simulink model "RL_SAC"  (R2025a)
settings: Solver=FixedStepDiscrete  StartTime=0.0  StopTime=20  FixedStep=1e-2  RelTol=1e-6
undefined symbols (not defined in the file or in its folder): DiscIntNeverNeededParam
libraries: simulink x26, cstblocks x16, slpidlib x2, aerolibutil x2, rllib x1
(part 2 of 2)

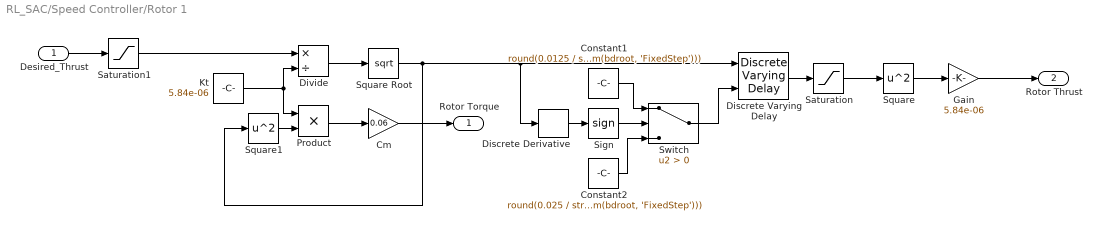
== system RL_SAC/Speed Controller/Rotor 1 ==
  Desired_Thrust : Inport
  Cm : Gain  Gain=0.06
  Constant1 : Constant  Value=round(0.0125 / str2double(get_param(bdroot, 'FixedStep')))
  Constant2 : Constant  Value=round(0.025 / str2double(get_param(bdroot, 'FixedStep')))
  Discrete Derivative : simulink/Discrete/Discrete Derivative  gainval=1.0  ICPrevScaledInput=0.0  OutMin=[]  OutMax=[]  OutDataType=fixdt(1, 16)  OutScaling=2^-10  DoSatur=off
  Discrete Varying Delay : cstblocks/Linear Parameter Varying/Discrete Varying Delay  Td=1  TdMax=10  TdFixed=[]  u0=0  Ts=-1  PreventDirectFeedthrough=off
  Divide : Product  Inputs=*/
  Gain : Gain  Gain=5.84e-06
  Kt : Constant  Value=5.84e-06
  Product : Product
  Saturation : Saturate  UpperLimit=1100  LowerLimit=0
  Saturation1 : Saturate  UpperLimit=inf  LowerLimit=0
  Sign : Signum
  Square : Math  Operator=square
  Square Root : Sqrt
  Square1 : Math  Operator=square
  Switch : Switch  Criteria=u2 > Threshold  SaturateOnIntegerOverflow=off  InputSameDT=off
  Rotor Torque : Outport
  Rotor Thrust : Outport  Port=2
  wires:
  Desired_Thrust/1 -> Saturation1/1
  Saturation/1 -> Square/1
  Switch/1 -> Discrete Varying Delay/2
  Constant2/1 -> Switch/3
  Discrete Varying Delay/1 -> Saturation/1
  Discrete Derivative/1 -> Sign/1
  Constant1/1 -> Switch/1
  Square Root/1 -> Discrete Varying Delay/1, Discrete Derivative/1, Square1/1
  Sign/1 -> Switch/2
  Square/1 -> Gain/1
  Kt/1 -> Divide/2, Product/1
  Divide/1 -> Square Root/1
  Product/1 -> Cm/1
  Square1/1 -> Product/2
  Cm/1 -> Rotor Torque/1
  Gain/1 -> Rotor Thrust/1
  Saturation1/1 -> Divide/1

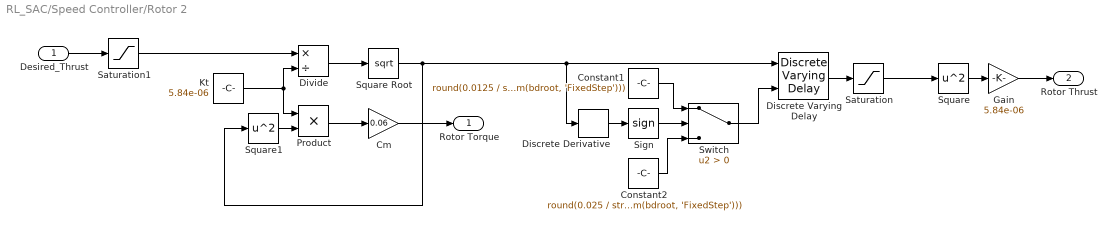
== system RL_SAC/Speed Controller/Rotor 2 ==
  Desired_Thrust : Inport
  Cm : Gain  Gain=0.06
  Constant1 : Constant  Value=round(0.0125 / str2double(get_param(bdroot, 'FixedStep')))
  Constant2 : Constant  Value=round(0.025 / str2double(get_param(bdroot, 'FixedStep')))
  Discrete Derivative : simulink/Discrete/Discrete Derivative  gainval=1.0  ICPrevScaledInput=0.0  OutMin=[]  OutMax=[]  OutDataType=fixdt(1, 16)  OutScaling=2^-10  DoSatur=off
  Discrete Varying Delay : cstblocks/Linear Parameter Varying/Discrete Varying Delay  Td=1  TdMax=10  TdFixed=[]  u0=0  Ts=-1  PreventDirectFeedthrough=off
  Divide : Product  Inputs=*/
  Gain : Gain  Gain=5.84e-06
  Kt : Constant  Value=5.84e-06
  Product : Product
  Saturation : Saturate  UpperLimit=1100  LowerLimit=0
  Saturation1 : Saturate  UpperLimit=inf  LowerLimit=0
  Sign : Signum
  Square : Math  Operator=square
  Square Root : Sqrt
  Square1 : Math  Operator=square
  Switch : Switch  Criteria=u2 > Threshold  SaturateOnIntegerOverflow=off  InputSameDT=off
  Rotor Torque : Outport
  Rotor Thrust : Outport  Port=2
  wires:
  Cm/1 -> Rotor Torque/1
  Square1/1 -> Product/2
  Product/1 -> Cm/1
  Divide/1 -> Square Root/1
  Kt/1 -> Product/1, Divide/2
  Saturation1/1 -> Divide/1
  Gain/1 -> Rotor Thrust/1
  Square/1 -> Gain/1
  Sign/1 -> Switch/2
  Square Root/1 -> Square1/1, Discrete Derivative/1, Discrete Varying Delay/1
  Constant1/1 -> Switch/1
  Discrete Derivative/1 -> Sign/1
  Discrete Varying Delay/1 -> Saturation/1
  Constant2/1 -> Switch/3
  Switch/1 -> Discrete Varying Delay/2
  Saturation/1 -> Square/1
  Desired_Thrust/1 -> Saturation1/1

== system RL_SAC/Speed Controller/Rotor 3 ==
  Desired_Thrust : Inport
  Cm : Gain  Gain=0.06
  Constant1 : Constant  Value=round(0.0125 / str2double(get_param(bdroot, 'FixedStep')))
  Constant2 : Constant  Value=round(0.025 / str2double(get_param(bdroot, 'FixedStep')))
  Discrete Derivative : simulink/Discrete/Discrete Derivative  gainval=1.0  ICPrevScaledInput=0.0  OutMin=[]  OutMax=[]  OutDataType=fixdt(1, 16)  OutScaling=2^-10  DoSatur=off
  Discrete Varying Delay : cstblocks/Linear Parameter Varying/Discrete Varying Delay  Td=1  TdMax=10  TdFixed=[]  u0=0  Ts=-1  PreventDirectFeedthrough=off
  Divide : Product  Inputs=*/
  Gain : Gain  Gain=5.84e-06
  Kt : Constant  Value=5.84e-06
  Product : Product
  Saturation : Saturate  UpperLimit=1100  LowerLimit=0
  Saturation1 : Saturate  UpperLimit=inf  LowerLimit=0
  Sign : Signum
  Square : Math  Operator=square
  Square Root : Sqrt
  Square1 : Math  Operator=square
  Switch : Switch  Criteria=u2 > Threshold  SaturateOnIntegerOverflow=off  InputSameDT=off
  Rotor Torque : Outport
  Rotor Thrust : Outport  Port=2
  wires:
  Desired_Thrust/1 -> Saturation1/1
  Saturation/1 -> Square/1
  Switch/1 -> Discrete Varying Delay/2
  Constant2/1 -> Switch/3
  Discrete Varying Delay/1 -> Saturation/1
  Discrete Derivative/1 -> Sign/1
  Constant1/1 -> Switch/1
  Square Root/1 -> Discrete Varying Delay/1, Discrete Derivative/1, Square1/1
  Sign/1 -> Switch/2
  Square/1 -> Gain/1
  Gain/1 -> Rotor Thrust/1
  Saturation1/1 -> Divide/1
  Kt/1 -> Divide/2, Product/1
  Divide/1 -> Square Root/1
  Product/1 -> Cm/1
  Square1/1 -> Product/2
  Cm/1 -> Rotor Torque/1

== system RL_SAC/Speed Controller/Rotor 4 ==
  Desired_Thrust : Inport
  Cm : Gain  Gain=0.06
  Constant1 : Constant  Value=round(0.0125 / str2double(get_param(bdroot, 'FixedStep')))
  Constant2 : Constant  Value=round(0.025 / str2double(get_param(bdroot, 'FixedStep')))
  Discrete Derivative : simulink/Discrete/Discrete Derivative  gainval=1.0  ICPrevScaledInput=0.0  OutMin=[]  OutMax=[]  OutDataType=fixdt(1, 16)  OutScaling=2^-10  DoSatur=off
  Discrete Varying Delay : cstblocks/Linear Parameter Varying/Discrete Varying Delay  Td=1  TdMax=10  TdFixed=[]  u0=0  Ts=-1  PreventDirectFeedthrough=off
  Divide : Product  Inputs=*/
  Gain : Gain  Gain=5.84e-06
  Kt : Constant  Value=5.84e-06
  Product : Product
  Saturation : Saturate  UpperLimit=1100  LowerLimit=0
  Saturation1 : Saturate  UpperLimit=inf  LowerLimit=0
  Sign : Signum
  Square : Math  Operator=square
  Square Root : Sqrt
  Square1 : Math  Operator=square
  Switch : Switch  Criteria=u2 > Threshold  SaturateOnIntegerOverflow=off  InputSameDT=off
  Rotor Torque : Outport
  Rotor Thrust : Outport  Port=2
  wires:
  Cm/1 -> Rotor Torque/1
  Square1/1 -> Product/2
  Product/1 -> Cm/1
  Divide/1 -> Square Root/1
  Kt/1 -> Product/1, Divide/2
  Saturation1/1 -> Divide/1
  Gain/1 -> Rotor Thrust/1
  Square/1 -> Gain/1
  Sign/1 -> Switch/2
  Square Root/1 -> Square1/1, Discrete Derivative/1, Discrete Varying Delay/1
  Constant1/1 -> Switch/1
  Discrete Derivative/1 -> Sign/1
  Discrete Varying Delay/1 -> Saturation/1
  Constant2/1 -> Switch/3
  Switch/1 -> Discrete Varying Delay/2
  Saturation/1 -> Square/1
  Desired_Thrust/1 -> Saturation1/1

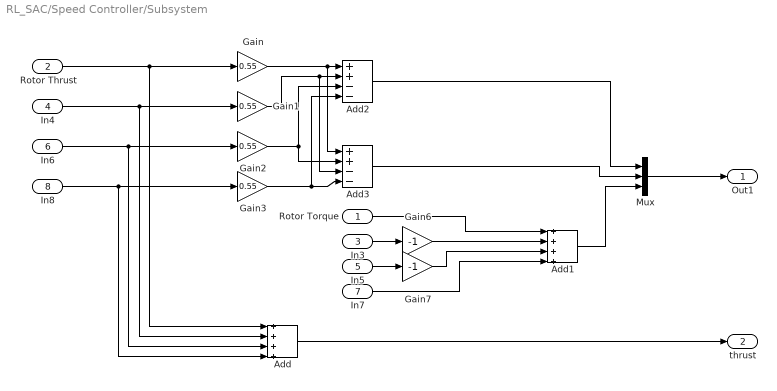
== system RL_SAC/Speed Controller/Subsystem ==
  Rotor Torque : Inport
  Rotor Thrust : Inport  Port=2
  In3 : Inport  Port=3
  In4 : Inport  Port=4
  In5 : Inport  Port=5
  In6 : Inport  Port=6
  In7 : Inport  Port=7
  In8 : Inport  Port=8
  Add : Sum  Inputs=++++
  Add1 : Sum  Inputs=++++
  Add2 : Sum  Inputs=++--
  Add3 : Sum  Inputs=++--
  Gain{,1..3} (4 alike) : Gain  Gain=0.55
  Gain6 : Gain  Gain=-1
  Gain7 : Gain  Gain=-1
  Mux : Mux  Inputs=3
  Out1 : Outport
  thrust : Outport  Port=2
  wires:
  Mux/1 -> Out1/1
  Add/1 -> thrust/1
  Add2/1 -> Mux/1
  Add3/1 -> Mux/2
  Add1/1 -> Mux/3
  In7/1 -> Add1/4
  In3/1 -> Gain6/1
  Rotor Torque/1 -> Add1/1
  In8/1 -> Gain3/1, Add/4
  Rotor Thrust/1 -> Gain/1, Add/1
  Gain/1 -> Add3/1, Add2/1
  Gain1/1 -> Add3/3, Add2/2
  Gain2/1 -> Add2/3, Add3/2
  Gain3/1 -> Add3/4, Add2/4
  In4/1 -> Add/2, Gain1/1
  In6/1 -> Add/3, Gain2/1
  Gain6/1 -> Add1/2
  In5/1 -> Gain7/1
  Gain7/1 -> Add1/3

== system RL_SAC/Attitude Control/RL/disturbance ==
  In1 : Inport
  DistDur : Inport  Port=2
  Add : Sum
  Add1 : Sum
  Constant : Constant  Value=6
  Delay : Delay  DelayLength=200
  Gain : Gain  Gain=-1
  Variable Time Delay : VariableTransportDelay  MaximumDelay=14  MaximumPoints=2048
  u : Outport
  wires:
  Gain/1 -> Variable Time Delay/1
  Delay/1 -> Add/1
  Variable Time Delay/1 -> Add/2
  In1/1 -> Delay/1, Gain/1
  Add/1 -> u/1
  Constant/1 -> Add1/2
  Add1/1 -> Variable Time Delay/2
  DistDur/1 -> Add1/1

== system RL_SAC/Attitude Control/RL/disturbance1 ==
  In1 : Inport
  DistDur : Inport  Port=2
  Add : Sum
  Add1 : Sum
  Constant : Constant  Value=2
  Delay : Delay  DelayLength=200
  Gain : Gain  Gain=-1
  Variable Time Delay : VariableTransportDelay  MaximumDelay=14  MaximumPoints=2048
  u : Outport
  wires:
  Add/1 -> u/1
  In1/1 -> Delay/1, Gain/1
  Variable Time Delay/1 -> Add/2
  Delay/1 -> Add/1
  Gain/1 -> Variable Time Delay/1
  Constant/1 -> Add1/2
  Add1/1 -> Variable Time Delay/2
  DistDur/1 -> Add1/1

== system RL_SAC/Attitude Control/RL/observation ==
  F_A_Pos : Inport
  b a vel : Inport  Port=2
  pos_error : Inport  Port=3
  DistDur : Inport  Port=4
  wind : Inport  Port=5
  Abs1 : Abs  SaturateOnIntegerOverflow=off
  Compare To Constant1 : simulink/Logic and Bit Operations/Compare To Constant  relop=>=  const=0.1  OutDataTypeStr=boolean
  Constant1 : Constant
  Data Type Conversion : DataTypeConversion  OutDataTypeStr=double  SaturateOnIntegerOverflow=off  RndMeth=Floor
  Mux : Mux  Inputs=5
  Selector2 : Selector  InputPortWidth=3  IndexOptions=Index vector (dialog)  Indices=[1]  OutputSizes=1
  disturbance1 : Subsystem
      settings: PortSchema="{\"entries\":[{\"content\":{\"sides\":[{\"content\":{\"connectorIds\":[\"In1\"]},\"type\":\"ConnectorPlacement.EquallySpacedRectSide\",\"uuid\":\"1ea45d97-72cc-4587-9cbf-0adeb2cc8bb7\"},{\"content\":{\"connectorIds\":[\"Out1\"],\"side\":\"RIGHT\"},\"type\":\"ConnectorPlacement.EquallySpacedRectSide\",\"uuid\":\"61165e1b-28cc-48e7-99ef-5ed7ad2a03a2\"},{\"content\":{\"side\":\"TOP\"},\"type\":\"ConnectorPlacement.EquallySpacedRectSide\",\"uuid\":\"1ee858fb-66c9-4560-b1d5-e0dc7ce4c9ca\"},{\"content\":{\"connectorIds\":[\"In2\"],\"side\":\"BOTTOM\"},\"type\":\"ConnectorPlacement.EquallySpacedRectSide\",\"uuid\":\"8aed40e2-8781-4923-8805-61cf0e1b563e\"}]},\"type\":\"ConnectorPlacement.EquallySpacedConnector\",\"uuid\":\"317ef023-ce87-4b82-add9-53b7146a0621\"}],\"packageUris\":[\"http://schema.mathworks.com/mf0/Connector/R2020b\"],\"version\":\"1.0\"}"
  Out1 : Outport
  wires:
  F_A_Pos/1 -> Selector2/1
  Abs1/1 -> Compare To Constant1/1
  Compare To Constant1/1 -> Data Type Conversion/1
  Data Type Conversion/1 -> Mux/2
  Mux/1 -> Out1/1
  Constant1/1 -> disturbance1/1(In1)
  disturbance1/1(u) -> Abs1/1
  DistDur/1 -> disturbance1/2(DistDur)
  wind/1 -> Mux/1
  Selector2/1 -> Mux/3
  b a vel/1 -> Mux/4
  pos_error/1 -> Mux/5

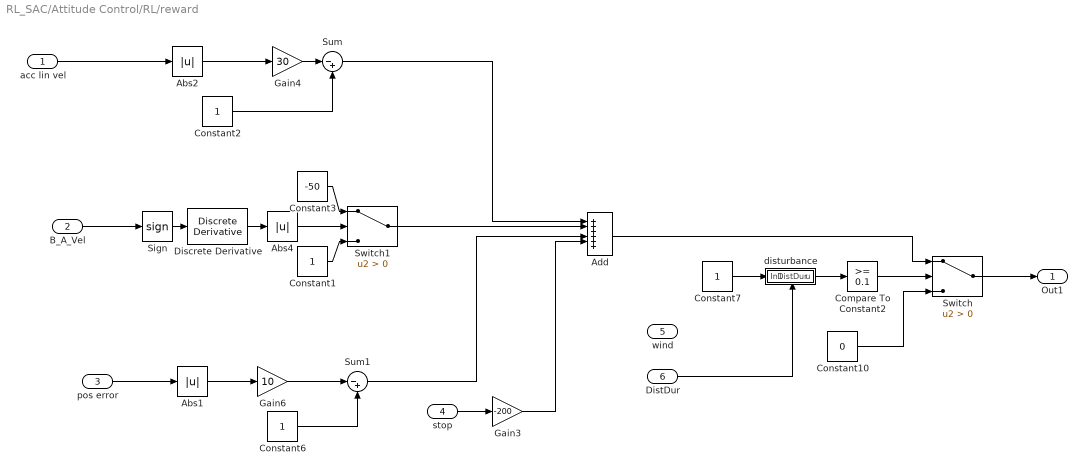
== system RL_SAC/Attitude Control/RL/reward ==
  acc lin vel : Inport
  B_A_Vel : Inport  Port=2
  pos error : Inport  Port=3
  stop : Inport  Port=4
  wind : Inport  Port=5
  DistDur : Inport  Port=6
  Abs1 : Abs  SaturateOnIntegerOverflow=off
  Abs2 : Abs  SaturateOnIntegerOverflow=off
  Abs4 : Abs  SaturateOnIntegerOverflow=off
  Add : Sum  Inputs=++++++
  Compare To Constant2 : simulink/Logic and Bit Operations/Compare To Constant  relop=>=  const=0.1  OutDataTypeStr=boolean
  Constant{1..2,6..7} (4 alike) : Constant
  Constant10 : Constant  Value=0
  Constant3 : Constant  Value=-50
  Discrete Derivative : simulink/Discrete/Discrete Derivative  gainval=1.0  ICPrevScaledInput=0.0  OutMin=[]  OutMax=[]  OutDataType=fixdt(1, 16)  OutScaling=2^-10  DoSatur=off
  Gain3 : Gain  Gain=-200
  Gain4 : Gain  Gain=30
  Gain6 : Gain  Gain=10
  Sign : Signum
  Sum : Sum  Inputs=|-+
  Sum1 : Sum  Inputs=|-+
  Switch : Switch  Criteria=u2 > Threshold  SaturateOnIntegerOverflow=off  InputSameDT=off
  Switch1 : Switch  Criteria=u2 > Threshold  SaturateOnIntegerOverflow=off  InputSameDT=off
  disturbance : Subsystem
      settings: PortSchema="{\"entries\":[{\"content\":{\"sides\":[{\"content\":{\"connectorIds\":[\"In1\"]},\"type\":\"ConnectorPlacement.EquallySpacedRectSide\",\"uuid\":\"1ea45d97-72cc-4587-9cbf-0adeb2cc8bb7\"},{\"content\":{\"connectorIds\":[\"Out1\"],\"side\":\"RIGHT\"},\"type\":\"ConnectorPlacement.EquallySpacedRectSide\",\"uuid\":\"61165e1b-28cc-48e7-99ef-5ed7ad2a03a2\"},{\"content\":{\"side\":\"TOP\"},\"type\":\"ConnectorPlacement.EquallySpacedRectSide\",\"uuid\":\"1ee858fb-66c9-4560-b1d5-e0dc7ce4c9ca\"},{\"content\":{\"connectorIds\":[\"In2\"],\"side\":\"BOTTOM\"},\"type\":\"ConnectorPlacement.EquallySpacedRectSide\",\"uuid\":\"88debdfa-6370-4c36-898f-2948795f08ca\"}]},\"type\":\"ConnectorPlacement.EquallySpacedConnector\",\"uuid\":\"317ef023-ce87-4b82-add9-53b7146a0621\"}],\"packageUris\":[\"http://schema.mathworks.com/mf0/Connector/R2020b\"],\"version\":\"1.0\"}"
  Out1 : Outport
  wires:
  Abs2/1 -> Gain4/1
  Constant10/1 -> Switch/3
  Abs1/1 -> Gain6/1
  stop/1 -> Gain3/1
  Sign/1 -> Discrete Derivative/1
  Discrete Derivative/1 -> Abs4/1
  Abs4/1 -> Switch1/2
  Constant1/1 -> Switch1/3
  Constant3/1 -> Switch1/1
  Switch1/1 -> Add/2
  Gain3/1 -> Add/5
  B_A_Vel/1 -> Sign/1
  Constant7/1 -> disturbance/1(In1)
  disturbance/1(u) -> Compare To Constant2/1
  Compare To Constant2/1 -> Switch/2
  Add/1 -> Switch/1
  Switch/1 -> Out1/1
  pos error/1 -> Abs1/1
  acc lin vel/1 -> Abs2/1
  Gain4/1 -> Sum/1
  Constant2/1 -> Sum/2
  Sum/1 -> Add/1
  Gain6/1 -> Sum1/1
  Sum1/1 -> Add/4
  Constant6/1 -> Sum1/2
  DistDur/1 -> disturbance/2(DistDur)

== system RL_SAC/Attitude Control/RL/stop ==
  pos error : Inport
  F_A_Pos : Inport  Port=2
  B_A_Vel : Inport  Port=3
  wind : Inport  Port=4
  DistDur : Inport  Port=5
  AND1 : Logic  IconShape=distinctive  AllPortsSameDT=off  OutDataTypeStr=boolean
  Abs : Abs  SaturateOnIntegerOverflow=off
  Abs2 : Abs  SaturateOnIntegerOverflow=off
  Abs3 : Abs  SaturateOnIntegerOverflow=off
  Compare To Constant : simulink/Logic and Bit Operations/Compare To Constant  relop=>=  const=2  OutDataTypeStr=boolean
  Compare To Constant1 : simulink/Logic and Bit Operations/Compare To Constant  relop=>=  const=0.1  OutDataTypeStr=boolean
  Compare To Constant2 : simulink/Logic and Bit Operations/Compare To Constant  relop=>=  const=2  OutDataTypeStr=boolean
  Compare To Constant3 : simulink/Logic and Bit Operations/Compare To Constant  relop=>=  const=1  OutDataTypeStr=boolean
  Constant7 : Constant
  OR1 : Logic  Operator=OR  IconShape=distinctive  AllPortsSameDT=off  OutDataTypeStr=boolean
  OR2 : Logic  Operator=OR  IconShape=distinctive  AllPortsSameDT=off  OutDataTypeStr=boolean
  Selector2 : Selector  InputPortWidth=3  IndexOptions=Index vector (dialog)  Indices=[1]  OutputSizes=1
  disturbance : Subsystem
      settings: PortSchema="{\"entries\":[{\"content\":{\"sides\":[{\"content\":{\"connectorIds\":[\"In1\"]},\"type\":\"ConnectorPlacement.EquallySpacedRectSide\",\"uuid\":\"1ea45d97-72cc-4587-9cbf-0adeb2cc8bb7\"},{\"content\":{\"connectorIds\":[\"Out1\"],\"side\":\"RIGHT\"},\"type\":\"ConnectorPlacement.EquallySpacedRectSide\",\"uuid\":\"61165e1b-28cc-48e7-99ef-5ed7ad2a03a2\"},{\"content\":{\"side\":\"TOP\"},\"type\":\"ConnectorPlacement.EquallySpacedRectSide\",\"uuid\":\"1ee858fb-66c9-4560-b1d5-e0dc7ce4c9ca\"},{\"content\":{\"connectorIds\":[\"In2\"],\"side\":\"BOTTOM\"},\"type\":\"ConnectorPlacement.EquallySpacedRectSide\",\"uuid\":\"86c6fb90-e8c6-48ee-82d5-b4d3db8632a5\"}]},\"type\":\"ConnectorPlacement.EquallySpacedConnector\",\"uuid\":\"317ef023-ce87-4b82-add9-53b7146a0621\"}],\"packageUris\":[\"http://schema.mathworks.com/mf0/Connector/R2020b\"],\"version\":\"1.0\"}"
  Out1 : Outport
  wires:
  Abs/1 -> Compare To Constant/1
  Compare To Constant/1 -> OR2/1
  Abs2/1 -> Compare To Constant2/1
  pos error/1 -> Abs/1
  B_A_Vel/1 -> Abs2/1
  Compare To Constant2/1 -> OR2/2
  Compare To Constant1/1 -> AND1/2
  AND1/1 -> Out1/1
  OR2/1 -> OR1/1
  Abs3/1 -> Compare To Constant3/1
  Selector2/1 -> Abs3/1
  F_A_Pos/1 -> Selector2/1
  Compare To Constant3/1 -> OR1/2
  OR1/1 -> AND1/1
  disturbance/1(u) -> Compare To Constant1/1
  DistDur/1 -> disturbance/2(DistDur)
  Constant7/1 -> disturbance/1(In1)

== system RL_SAC/Gyro/noise/Subsystem1 ==
  "  " : Inport
  Selector : Selector  InputPortWidth=3  IndexOptions=Index vector (dialog)  Indices=[1]  OutputSizes=1
  Selector1 : Selector  InputPortWidth=3  IndexOptions=Index vector (dialog)  Indices=[2]  OutputSizes=1
  Selector2 : Selector  InputPortWidth=3  IndexOptions=Index vector (dialog)  Indices=[3]  OutputSizes=1
  Out1 : Outport
  Out2 : Outport  Port=2
  Out3 : Outport  Port=3
  wires:
  Selector2/1 -> Out3/1
  Selector1/1 -> Out2/1
  Selector/1 -> Out1/1
  "  "/1 -> Selector2/1, Selector/1, Selector1/1

== system RL_SAC/Position Control/Subsystem3/Subsystem1 ==
  u : Inport
  Abs1 : Abs  SaturateOnIntegerOverflow=off
  MATLAB Function : MATLAB Function  TreatAsAtomicUnit=on
  y : Outport
  wires:
  MATLAB Function/1(y) -> y/1
  u/1 -> Abs1/1
  Abs1/1 -> MATLAB Function/1(u)

== system RL_SAC/Position Control/Subsystem3/Subsystem5 ==
  u : Inport
  Abs1 : Abs  SaturateOnIntegerOverflow=off
  MATLAB Function : MATLAB Function  TreatAsAtomicUnit=on
  y : Outport
  wires:
  MATLAB Function/1(y) -> y/1
  u/1 -> Abs1/1
  Abs1/1 -> MATLAB Function/1(u)

== system RL_SAC/Position Control/Subsystem4/Subsystem1 ==
  u : Inport
  Abs1 : Abs  SaturateOnIntegerOverflow=off
  MATLAB Function : MATLAB Function  TreatAsAtomicUnit=on
  y : Outport
  wires:
  MATLAB Function/1(y) -> y/1
  u/1 -> Abs1/1
  Abs1/1 -> MATLAB Function/1(u)

== system RL_SAC/Position Control/Subsystem4/Subsystem2 ==
  u : Inport
  Abs1 : Abs  SaturateOnIntegerOverflow=off
  MATLAB Function : MATLAB Function  TreatAsAtomicUnit=on
  y : Outport
  wires:
  Abs1/1 -> MATLAB Function/1(u)
  MATLAB Function/1(y) -> y/1
  u/1 -> Abs1/1

== system RL_SAC/Attitude Control/RL/observation/disturbance1 ==
  In1 : Inport
  DistDur : Inport  Port=2
  Add : Sum
  Add1 : Sum
  Constant : Constant  Value=6
  Delay : Delay  DelayLength=100  SampleTime=1e-2
  Gain : Gain  Gain=-1
  Variable Time Delay : VariableTransportDelay  MaximumDelay=14  MaximumPoints=2048
  u : Outport
  wires:
  Add/1 -> u/1
  In1/1 -> Gain/1, Delay/1
  Variable Time Delay/1 -> Add/2
  Delay/1 -> Add/1
  Gain/1 -> Variable Time Delay/1
  Constant/1 -> Add1/2
  Add1/1 -> Variable Time Delay/2
  DistDur/1 -> Add1/1

== system RL_SAC/Attitude Control/RL/reward/disturbance ==
  In1 : Inport
  DistDur : Inport  Port=2
  Add : Sum
  Add1 : Sum
  Constant : Constant  Value=6
  Delay : Delay  DelayLength=200
  Gain : Gain  Gain=-1
  Variable Time Delay : VariableTransportDelay  MaximumDelay=14  MaximumPoints=2048
  u : Outport
  wires:
  Gain/1 -> Variable Time Delay/1
  Delay/1 -> Add/1
  Variable Time Delay/1 -> Add/2
  In1/1 -> Delay/1, Gain/1
  Add/1 -> u/1
  Constant/1 -> Add1/2
  Add1/1 -> Variable Time Delay/2
  DistDur/1 -> Add1/1

== system RL_SAC/Attitude Control/RL/stop/disturbance ==
  In1 : Inport
  DistDur : Inport  Port=2
  Add : Sum
  Add1 : Sum
  Constant : Constant  Value=6
  Delay : Delay  DelayLength=200
  Gain : Gain  Gain=-1
  Variable Time Delay : VariableTransportDelay  MaximumDelay=14  MaximumPoints=2048
  u : Outport
  wires:
  Gain/1 -> Variable Time Delay/1
  Delay/1 -> Add/1
  Variable Time Delay/1 -> Add/2
  In1/1 -> Delay/1, Gain/1
  Add/1 -> u/1
  Constant/1 -> Add1/2
  Add1/1 -> Variable Time Delay/2
  DistDur/1 -> Add1/1

== matlab function RL_SAC/Dynamic Model/MATLAB Function1 ==
  data: a output; torque input; thrust input; qdlin input; qdang input; qang input; wind input
function a = dynamics(torque, thrust, qdlin, qdang, qang, wind)
% torth = [Xtor; Ytor; Ztor; thrusttot];
%% Drone Parameters
MassD = 1.282; % Mass of Drone - Kg
g = 9.81; % Acceleration due to gravity - m/s^2
gref = [0; 0; -g]; % gravity in reference frame
rho = 1.225; % air density amsl kgm-3

etad = [qang(1); qang(2); qang(3)]; % rotation
eta = [deg2rad(etad(1)); deg2rad(etad(2)); deg2rad(etad(3))]; % rotation
vel = [qdlin(1); qdlin(2); qdlin(3)]; % uav velocity ms-1
RelWin = -vel + wind; % relative airspeed caused by movement through air
Fi = [0;0;thrust]; % Thrust
%% Rotation matrix
Rgx = [1 0      0;
      0 cos(eta(1))  sin(eta(1));
      0 -sin(eta(1)) cos(eta(1))];
Rgy = [cos(eta(2)) 0 sin(eta(2));
      0           1 0;
      -sin(eta(2)) 0 cos(eta(2))];
Rgz = [cos(eta(3)) -sin(eta(3)) 0;
      sin(eta(3)) cos(eta(3))  0;
      0           0            1];
RotBtR = Rgz*Rgy*Rgx; % body to reference frame rotation
%% inertia matrix
ixx = 0.029125;
iyy = 0.029125;
izz = 0.055225;
I = diag([ixx, iyy, izz]);
%% Gravity force matrix
Fg = (RotBtR'*gref); % gravitational acceleration (xyz) in body frame
Fgf = Fg*MassD; % gravitational force (xyz) in body frame
%% Drag force
%linear
cdyi = 0.1150546; % cd at 0ms-1
cdm = 5.8454e-3; % cd multiplier (gradient for cd/speed)
%Cdlin = [cdyi+(cdm*qdlin(1));cdyi+(cdm*qdlin(2)) ;cdyi+(cdm*qdlin(3)) ]; % Coefficient of drage estimate
Cdlin = [0.1;0.1;0.1];


WArea = [0.017; 0.014; 0.047]; % Wind facing area estimate m^2 - from 3d model (y is front)
Fd = [0.5*rho*Cdlin(1)*WArea(1)*(RelWin(1)^2); 0.5*rho*Cdlin(2)*WArea(2)*(RelWin(2)^2); 0.5*rho*Cdlin(3)*WArea(3)*(RelWin(3)^2)]; % Drag Force matrix
%rotation
Cdrot = [cdyi+(cdm*qdang(1));cdyi+(cdm*qdang(2)) ;cdyi+(cdm*qdang(3)) ];
RArea = [0.047;0.047;0.012];
Cti = [0.5*rho*RArea(1)*Cdrot(1);0.5*rho*RArea(2)*Cdrot(2);0.5*rho*RArea(3)*Cdrot(3)];
Taudr = [(qdang(1)^2)*Cti(1); (qdang(2)^2)*Cti(2); (qdang(3)^2)*Cti(3)];
if qdang(1) > 0 
    Taudr(1) = -Taudr(1);
else
    Taudr(1) = Taudr(1);
end
if qdang(2) > 0
    Taudr(2) = -Taudr(2);
else
    Taudr(2) = Taudr(2);
end
if qdang(3) > 0
    Taudr(3) = -Taudr(3);
else
    Taudr(3) = Taudr(3);
end
%% acceleration
% linear acceleration
abx = (Fgf(1)+Fd(1))/MassD; % body x axis acceleration
aby = (Fgf(2)+Fd(2))/MassD; % body y axis acceleration
abz = (Fi(3) + Fgf(3) + Fd(3))/MassD; % body z axis acceleration
alinb = [abx; aby; abz];
alinr = RotBtR*alinb; % body to reference frame conversion
alin = [alinb(1); alinb(2); alinb(3); alinr(1); alinr(2); alinr(3);]; % linear acceleration - [body frame ; ref frame]
% angular acceleration
tau = [torque(1)+Taudr(1); torque(2)+Taudr(2); torque(3)+Taudr(3)];
vrotb = [qdang(1); qdang(2); qdang(3)];

arotb = I \ (tau - cross(vrotb, I*vrotb)); %[ixx*tau(1);iyy*tau(2);izz*tau(3)]; 
arotr = RotBtR*arotb;
arot = [arotb(1); arotb(2); arotb(3); arotr(1); arotr(2); arotr(3);]; %rotational acceleration

a = [alin; arot];

end

== matlab function RL_SAC/Position Control/Subsystem4/Subsystem2/MATLAB Function ==
  data: u input; y output
function y = fcn(u)
a = 0;
if u < 0.4
    a = 15;
end
if u <= 1 && u >= 0.4
    a = 8*(u^-0.686);
end
if u > 1
    a = 8;
end

y = a;

== matlab function RL_SAC/Position Control/Subsystem6/MATLAB Function ==
  data: u input; y output
function y = fcn(u)
a = 0;
if u <= 0.4
    a = 0.5;
end
if u > 0.4
    a = 0.3392*(u^-0.317);
end

y = a;

== matlab function RL_SAC/Attitude Control/Quaternion P control/MATLAB Function ==
  data: eul input; quat output
function quat = eulTOquat(eul)
eulv = [eul(1) eul(2) eul(3)];
quatr = eul2quat(eulv, 'XYZ');
quat = quatr(:);
end

== matlab function RL_SAC/Attitude Control/Quaternion P control/MATLAB Function1 ==
  data: eul input; quat output
function quat = eulTOquat(eul)
eulv = [eul(1) eul(2) eul(3)];
quatr = eul2quat(eulv, 'XYZ');
quat = quatr(:);
end

== matlab function RL_SAC/Position Control/Subsystem3/Subsystem5/MATLAB Function ==
  data: u input; y output
function y = fcn(u)
a = 0;
if u < 0.4
    a = 15;
end
if u <= 1 && u >= 0.4
    a = 8*(u^-0.686);
end
if u > 1
    a = 8;
end

y = a;

== matlab function RL_SAC/Position Control/Subsystem3/Subsystem1/MATLAB Function ==
  data: u input; y output
function y = fcn(u)
a = 0;
if u < 0.4
    a = 6;
end
if u <= 15 && u >= 0.4
    a = 5.3592*(u^-0.094);
end
if u > 15
    a = 4;
end

y = a;

== matlab function RL_SAC/Position Control/Subsystem4/Subsystem1/MATLAB Function ==
  data: u input; y output
function y = fcn(u)
a = 0;
if u < 0.4
    a = 6;
end
if u <= 15 && u >= 0.4
    a = 5.3592*(u^-0.094);
end
if u > 15
    a = 4;
end

y = a;

== matlab function RL_SAC/Position Control/Subsystem5/MATLAB Function ==
  data: u input; y output
function y = fcn(u)
a = 0;
if u <= 0.4
    a = 0.5;
end
if u > 0.4
    a = 0.3392*(u^-0.317);
end

y = a;
